simulink model "dq_model"  (R2015a)
settings: Solver=ode45  StartTime=0.0  StopTime=1.5  FixedStep=1e-5  MaxStep=1e-3  RelTol=1e-3
InitFcn:
  | parametriAM
values from neighbouring files (symbols this model uses):
  Imrn = 7.4    [parametriAM.m]
  Ismax = In*sqrt(2)    [parametriAM.m]
  J = 0.019    [parametriAM.m]    (also in podatki.m = 0.01)
  Ki_Imr = 1000    [parametriAM.m]
  Ki_tok = 5.0    (= 5)    [parametriAM.m]
  Ki_wr = 1000    [parametriAM.m]
  Kp_Imr = 100    [parametriAM.m]
  Kp_tok = 0.05    [parametriAM.m]
  Kp_wr = 50    [parametriAM.m]
  Lm = 0.0493    [parametriAM.m]    (also in podatki.m = 0.2342)
  Lr = 0.05315    [parametriAM.m]    (also in podatki.m = 0.2449)
  Ls = 0.05315    [parametriAM.m]    (also in podatki.m = 0.2449)
  Lst = sigma*Ls    (= 0.00742111947319)    [parametriAM.m]
  pp = 3    [parametriAM.m]    (also in podatki.m = 2)
  Rs = 0.594    [parametriAM.m]    (also in podatki.m = 3.7)
  sigma = 1 - 1/((1+sigmaR)*(1+sigmaS))    (= 0.13962595434)    [parametriAM.m]
  Tr = Lr/Rr    (= 0.0771407837446)    [parametriAM.m]
  Udc = Un*sqrt(2)    [parametriAM.m]
  wb_upper_limit_field_weaking = sqrt((Ls^2+Lst^2)/(2*Lst^2*Ls^2))*Usmax/Ismax    [parametriAM.m]
  wn = Udc/sqrt(Ls^2*(Imrn)^2+Lst^2*(Ismax^2-(Imrn)^2))    [maximalnaelipsa.m]    (also in parametriAM.m = Un/sqrt(Ls^2*(Imrn)^2+Lst^2*(Ismax^2-(Imrn)^2))/pp)
libraries: simulink x20
(part 2 of 2)

== system dq_model/motor/Transformacije/Inverzni Park ==
  kot : Inport
  U_dq : Inport  Port=2
  Demux : Demux  Outputs=2
  Mux : Mux  Inputs=2
  "Sum1 " : Sum  Inputs=+-  SaturateOnIntegerOverflow=on  InputSameDT=on  OutDataTypeStr=Inherit: Same as first input
  Sum2 : Sum  SaturateOnIntegerOverflow=on  InputSameDT=on  OutDataTypeStr=Inherit: Same as first input
  cos : Fcn  Expr=cos(u)
  sin : Fcn  Expr=sin(u)
  x_d*cos : Product  SaturateOnIntegerOverflow=on  RndMeth=Zero  InputSameDT=on  OutDataTypeStr=Inherit: Same as first input
  x_d*sin : Product  SaturateOnIntegerOverflow=on  RndMeth=Zero  InputSameDT=on  OutDataTypeStr=Inherit: Same as first input
  x_q*cos : Product  SaturateOnIntegerOverflow=on  RndMeth=Zero  InputSameDT=on  OutDataTypeStr=Inherit: Same as first input
  "x_q*sin " : Product  SaturateOnIntegerOverflow=on  RndMeth=Zero  InputSameDT=on  OutDataTypeStr=Inherit: Same as first input
  U_ab : Outport
  wires:
  Mux/1 -> U_ab/1
  U_dq/1 -> Demux/1
  Demux/1 -> x_d*sin/1, x_d*cos/1
  Demux/2 -> "x_q*sin "/1, x_q*cos/1
  cos/1 -> x_q*cos/2, x_d*cos/2
  sin/1 -> "x_q*sin "/2, x_d*sin/2
  x_d*cos/1 -> "Sum1 "/1
  "x_q*sin "/1 -> "Sum1 "/2
  x_q*cos/1 -> Sum2/2
  x_d*sin/1 -> Sum2/1
  "Sum1 "/1 -> Mux/1
  Sum2/1 -> Mux/2
  kot/1 -> cos/1, sin/1

== system dq_model/motor1/Asinhronski stroj1/Clarke ==
  U_123 : Inport
  ABC_ab1 : Subsystem
  Demux : Demux  Outputs=3
  Mux : Mux  Inputs=2
  U_ab : Outport
  wires:
  U_123/1 -> Demux/1
  Demux/1 -> ABC_ab1/1(A)
  Demux/2 -> ABC_ab1/2(B)
  Demux/3 -> ABC_ab1/3(C)
  ABC_ab1/1(alfa) -> Mux/1
  ABC_ab1/2(beta) -> Mux/2
  Mux/1 -> U_ab/1

== system dq_model/motor1/Asinhronski stroj1/Inverzni Clarke ==
  I_ab : Inport
  Demux : Demux  Outputs=2
  Mux : Mux  Inputs=3
  ab_ABC : Subsystem
  I_123 : Outport
  wires:
  Mux/1 -> I_123/1
  I_ab/1 -> Demux/1
  Demux/1 -> ab_ABC/1(alfa)
  Demux/2 -> ab_ABC/2(beta)
  ab_ABC/1(A) -> Mux/1
  ab_ABC/2(B) -> Mux/2
  ab_ABC/3(C) -> Mux/3

== system dq_model/motor1/Asinhronski stroj1/Inverzni Park ==
  I_dq : Inport
  kot : Inport  Port=2
  Demux : Demux  Outputs=2
  Mux : Mux  Inputs=2
  "Sum1 " : Sum  Inputs=+-  SaturateOnIntegerOverflow=on  InputSameDT=on  OutDataTypeStr=Inherit: Same as first input
  Sum2 : Sum  SaturateOnIntegerOverflow=on  InputSameDT=on  OutDataTypeStr=Inherit: Same as first input
  cos : Fcn  Expr=cos(u)
  sin : Fcn  Expr=sin(u)
  x_d*cos : Product  SaturateOnIntegerOverflow=on  RndMeth=Zero  InputSameDT=on  OutDataTypeStr=Inherit: Same as first input
  x_d*sin : Product  SaturateOnIntegerOverflow=on  RndMeth=Zero  InputSameDT=on  OutDataTypeStr=Inherit: Same as first input
  x_q*cos : Product  SaturateOnIntegerOverflow=on  RndMeth=Zero  InputSameDT=on  OutDataTypeStr=Inherit: Same as first input
  "x_q*sin " : Product  SaturateOnIntegerOverflow=on  RndMeth=Zero  InputSameDT=on  OutDataTypeStr=Inherit: Same as first input
  I_ab : Outport
  wires:
  kot/1 -> sin/1, cos/1
  Sum2/1 -> Mux/2
  "Sum1 "/1 -> Mux/1
  x_d*sin/1 -> Sum2/1
  x_q*cos/1 -> Sum2/2
  "x_q*sin "/1 -> "Sum1 "/2
  x_d*cos/1 -> "Sum1 "/1
  sin/1 -> x_d*sin/2, "x_q*sin "/2
  cos/1 -> x_d*cos/2, x_q*cos/2
  Demux/2 -> x_q*cos/1, "x_q*sin "/1
  Demux/1 -> x_d*cos/1, x_d*sin/1
  I_dq/1 -> Demux/1
  Mux/1 -> I_ab/1

== system dq_model/motor1/Asinhronski stroj1/Mehanika ==
  M_br : Inport
  M_el : Inport  Port=2
  Sum : Sum  Inputs=+-
  eq 2.19 : Subsystem
  wr : Outport
  wires:
  eq 2.19/1(wr) -> wr/1
  M_el/1 -> Sum/1
  Sum/1 -> eq 2.19/1(M)
  M_br/1 -> Sum/2

== system dq_model/motor1/Asinhronski stroj1/Park ==
  U_ab : Inport
  kot : Inport  Port=2
  Demux : Demux  Outputs=2
  Mux : Mux  Inputs=2
  "Sum1 " : Sum  SaturateOnIntegerOverflow=on  InputSameDT=on  OutDataTypeStr=Inherit: Same as first input
  Sum2 : Sum  Inputs=-+  SaturateOnIntegerOverflow=on  InputSameDT=on  OutDataTypeStr=Inherit: Same as first input
  cos : Fcn  Expr=cos(u)
  sin : Fcn  Expr=sin(u)
  x_a*cos : Product  SaturateOnIntegerOverflow=on  RndMeth=Zero  InputSameDT=on  OutDataTypeStr=Inherit: Same as first input
  x_a*sin : Product  SaturateOnIntegerOverflow=on  RndMeth=Zero  InputSameDT=on  OutDataTypeStr=Inherit: Same as first input
  x_b*cos : Product  SaturateOnIntegerOverflow=on  RndMeth=Zero  InputSameDT=on  OutDataTypeStr=Inherit: Same as first input
  "x_b*sin " : Product  SaturateOnIntegerOverflow=on  RndMeth=Zero  InputSameDT=on  OutDataTypeStr=Inherit: Same as first input
  U_dq : Outport
  wires:
  kot/1 -> sin/1, cos/1
  Sum2/1 -> Mux/2
  "Sum1 "/1 -> Mux/1
  x_a*sin/1 -> Sum2/1
  x_b*cos/1 -> Sum2/2
  "x_b*sin "/1 -> "Sum1 "/2
  x_a*cos/1 -> "Sum1 "/1
  sin/1 -> x_a*sin/2, "x_b*sin "/2
  cos/1 -> x_a*cos/2, x_b*cos/2
  Demux/2 -> x_b*cos/1, "x_b*sin "/1
  Demux/1 -> x_a*cos/1, x_a*sin/1
  U_ab/1 -> Demux/1
  Mux/1 -> U_dq/1

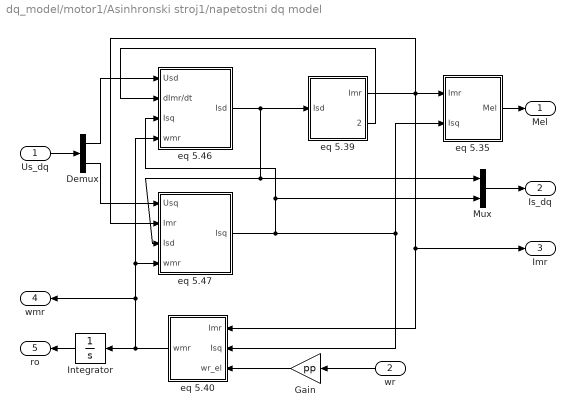
== system dq_model/motor1/Asinhronski stroj1/napetostni dq model ==
  Us_dq : Inport
  wr : Inport  Port=2
  Demux : Demux  Outputs=2
  Gain : Gain  Gain=pp
  Integrator : Integrator
  Mux : Mux  Inputs=2
  eq 5.35 : Subsystem
  eq 5.39 : Subsystem
  eq 5.40 : Subsystem
  eq 5.46 : Subsystem
  eq 5.47 : Subsystem
  Mel : Outport
  Is_dq : Outport  Port=2
  Imr : Outport  Port=3
  wmr : Outport  Port=4
  ro : Outport  Port=5
  wires:
  eq 5.46/1(Isd) -> eq 5.39/1(Isd), eq 5.47/3(Isd), Mux/1
  eq 5.39/2(dImr/dt) -> eq 5.46/2(dImr/dt)
  eq 5.39/1(Imr) -> eq 5.35/1(Imr), eq 5.40/1(Imr), Imr/1, eq 5.47/2(Imr)
  eq 5.47/1(Isq) -> eq 5.35/2(Isq), eq 5.40/2(Isq), eq 5.46/3(Isq), Mux/2
  eq 5.40/1(wmr) -> eq 5.47/4(wmr), eq 5.46/4(wmr), wmr/1, Integrator/1
  eq 5.35/1(Mel) -> Mel/1
  Integrator/1 -> ro/1
  wr/1 -> Gain/1
  Us_dq/1 -> Demux/1
  Demux/1 -> eq 5.46/1(Usd)
  Demux/2 -> eq 5.47/1(Usq)
  Mux/1 -> Is_dq/1
  Gain/1 -> eq 5.40/3(wr_el)

== system dq_model/motor1/Transformacije/Inverzni Clarke ==
  U_ab : Inport
  Demux : Demux  Outputs=2
  Mux : Mux  Inputs=3
  ab_ABC : Subsystem
  U_123 : Outport
  wires:
  Mux/1 -> U_123/1
  U_ab/1 -> Demux/1
  Demux/1 -> ab_ABC/1(alfa)
  Demux/2 -> ab_ABC/2(beta)
  ab_ABC/1(A) -> Mux/1
  ab_ABC/2(B) -> Mux/2
  ab_ABC/3(C) -> Mux/3

== system dq_model/motor1/Transformacije/Inverzni Park ==
  kot : Inport
  U_dq : Inport  Port=2
  Demux : Demux  Outputs=2
  Mux : Mux  Inputs=2
  "Sum1 " : Sum  Inputs=+-  SaturateOnIntegerOverflow=on  InputSameDT=on  OutDataTypeStr=Inherit: Same as first input
  Sum2 : Sum  SaturateOnIntegerOverflow=on  InputSameDT=on  OutDataTypeStr=Inherit: Same as first input
  cos : Fcn  Expr=cos(u)
  sin : Fcn  Expr=sin(u)
  x_d*cos : Product  SaturateOnIntegerOverflow=on  RndMeth=Zero  InputSameDT=on  OutDataTypeStr=Inherit: Same as first input
  x_d*sin : Product  SaturateOnIntegerOverflow=on  RndMeth=Zero  InputSameDT=on  OutDataTypeStr=Inherit: Same as first input
  x_q*cos : Product  SaturateOnIntegerOverflow=on  RndMeth=Zero  InputSameDT=on  OutDataTypeStr=Inherit: Same as first input
  "x_q*sin " : Product  SaturateOnIntegerOverflow=on  RndMeth=Zero  InputSameDT=on  OutDataTypeStr=Inherit: Same as first input
  U_ab : Outport
  wires:
  kot/1 -> sin/1, cos/1
  Sum2/1 -> Mux/2
  "Sum1 "/1 -> Mux/1
  x_d*sin/1 -> Sum2/1
  x_q*cos/1 -> Sum2/2
  "x_q*sin "/1 -> "Sum1 "/2
  x_d*cos/1 -> "Sum1 "/1
  sin/1 -> x_d*sin/2, "x_q*sin "/2
  cos/1 -> x_d*cos/2, x_q*cos/2
  Demux/2 -> x_q*cos/1, "x_q*sin "/1
  Demux/1 -> x_d*cos/1, x_d*sin/1
  U_dq/1 -> Demux/1
  Mux/1 -> U_ab/1

== system dq_model/motor2/Asinhronski stroj1/Clarke ==
  U_123 : Inport
  ABC_ab1 : Subsystem
  Demux : Demux  Outputs=3
  Mux : Mux  Inputs=2
  U_ab : Outport
  wires:
  Mux/1 -> U_ab/1
  ABC_ab1/2(beta) -> Mux/2
  ABC_ab1/1(alfa) -> Mux/1
  Demux/3 -> ABC_ab1/3(C)
  Demux/2 -> ABC_ab1/2(B)
  Demux/1 -> ABC_ab1/1(A)
  U_123/1 -> Demux/1

== system dq_model/motor2/Asinhronski stroj1/Inverzni Clarke ==
  I_ab : Inport
  Demux : Demux  Outputs=2
  Mux : Mux  Inputs=3
  ab_ABC : Subsystem
  I_123 : Outport
  wires:
  ab_ABC/3(C) -> Mux/3
  ab_ABC/2(B) -> Mux/2
  ab_ABC/1(A) -> Mux/1
  Demux/2 -> ab_ABC/2(beta)
  Demux/1 -> ab_ABC/1(alfa)
  I_ab/1 -> Demux/1
  Mux/1 -> I_123/1

== system dq_model/motor2/Asinhronski stroj1/Inverzni Park ==
  I_dq : Inport
  kot : Inport  Port=2
  Demux : Demux  Outputs=2
  Mux : Mux  Inputs=2
  "Sum1 " : Sum  Inputs=+-  SaturateOnIntegerOverflow=on  InputSameDT=on  OutDataTypeStr=Inherit: Same as first input
  Sum2 : Sum  SaturateOnIntegerOverflow=on  InputSameDT=on  OutDataTypeStr=Inherit: Same as first input
  cos : Fcn  Expr=cos(u)
  sin : Fcn  Expr=sin(u)
  x_d*cos : Product  SaturateOnIntegerOverflow=on  RndMeth=Zero  InputSameDT=on  OutDataTypeStr=Inherit: Same as first input
  x_d*sin : Product  SaturateOnIntegerOverflow=on  RndMeth=Zero  InputSameDT=on  OutDataTypeStr=Inherit: Same as first input
  x_q*cos : Product  SaturateOnIntegerOverflow=on  RndMeth=Zero  InputSameDT=on  OutDataTypeStr=Inherit: Same as first input
  "x_q*sin " : Product  SaturateOnIntegerOverflow=on  RndMeth=Zero  InputSameDT=on  OutDataTypeStr=Inherit: Same as first input
  I_ab : Outport
  wires:
  Mux/1 -> I_ab/1
  I_dq/1 -> Demux/1
  Demux/1 -> x_d*sin/1, x_d*cos/1
  Demux/2 -> "x_q*sin "/1, x_q*cos/1
  cos/1 -> x_q*cos/2, x_d*cos/2
  sin/1 -> "x_q*sin "/2, x_d*sin/2
  x_d*cos/1 -> "Sum1 "/1
  "x_q*sin "/1 -> "Sum1 "/2
  x_q*cos/1 -> Sum2/2
  x_d*sin/1 -> Sum2/1
  "Sum1 "/1 -> Mux/1
  Sum2/1 -> Mux/2
  kot/1 -> cos/1, sin/1

== system dq_model/motor2/Asinhronski stroj1/Mehanika ==
  M_br : Inport
  M_el : Inport  Port=2
  Sum : Sum  Inputs=+-
  eq 2.19 : Subsystem
  wr : Outport
  wires:
  M_br/1 -> Sum/2
  Sum/1 -> eq 2.19/1(M)
  M_el/1 -> Sum/1
  eq 2.19/1(wr) -> wr/1

== system dq_model/motor2/Asinhronski stroj1/Park ==
  U_ab : Inport
  kot : Inport  Port=2
  Demux : Demux  Outputs=2
  Mux : Mux  Inputs=2
  "Sum1 " : Sum  SaturateOnIntegerOverflow=on  InputSameDT=on  OutDataTypeStr=Inherit: Same as first input
  Sum2 : Sum  Inputs=-+  SaturateOnIntegerOverflow=on  InputSameDT=on  OutDataTypeStr=Inherit: Same as first input
  cos : Fcn  Expr=cos(u)
  sin : Fcn  Expr=sin(u)
  x_a*cos : Product  SaturateOnIntegerOverflow=on  RndMeth=Zero  InputSameDT=on  OutDataTypeStr=Inherit: Same as first input
  x_a*sin : Product  SaturateOnIntegerOverflow=on  RndMeth=Zero  InputSameDT=on  OutDataTypeStr=Inherit: Same as first input
  x_b*cos : Product  SaturateOnIntegerOverflow=on  RndMeth=Zero  InputSameDT=on  OutDataTypeStr=Inherit: Same as first input
  "x_b*sin " : Product  SaturateOnIntegerOverflow=on  RndMeth=Zero  InputSameDT=on  OutDataTypeStr=Inherit: Same as first input
  U_dq : Outport
  wires:
  Mux/1 -> U_dq/1
  U_ab/1 -> Demux/1
  Demux/1 -> x_a*sin/1, x_a*cos/1
  Demux/2 -> "x_b*sin "/1, x_b*cos/1
  cos/1 -> x_b*cos/2, x_a*cos/2
  sin/1 -> "x_b*sin "/2, x_a*sin/2
  x_a*cos/1 -> "Sum1 "/1
  "x_b*sin "/1 -> "Sum1 "/2
  x_b*cos/1 -> Sum2/2
  x_a*sin/1 -> Sum2/1
  "Sum1 "/1 -> Mux/1
  Sum2/1 -> Mux/2
  kot/1 -> cos/1, sin/1

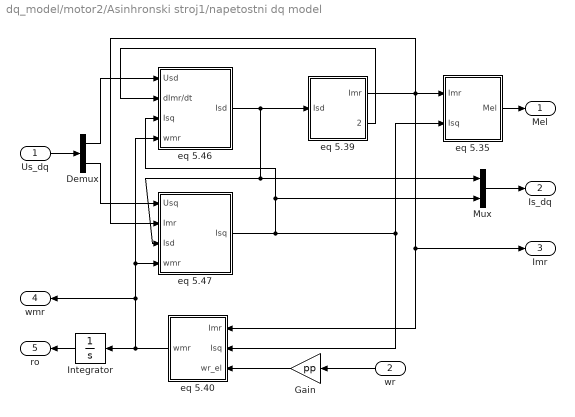
== system dq_model/motor2/Asinhronski stroj1/napetostni dq model ==
  Us_dq : Inport
  wr : Inport  Port=2
  Demux : Demux  Outputs=2
  Gain : Gain  Gain=pp
  Integrator : Integrator
  Mux : Mux  Inputs=2
  eq 5.35 : Subsystem
  eq 5.39 : Subsystem
  eq 5.40 : Subsystem
  eq 5.46 : Subsystem
  eq 5.47 : Subsystem
  Mel : Outport
  Is_dq : Outport  Port=2
  Imr : Outport  Port=3
  wmr : Outport  Port=4
  ro : Outport  Port=5
  wires:
  Gain/1 -> eq 5.40/3(wr_el)
  Mux/1 -> Is_dq/1
  Demux/2 -> eq 5.47/1(Usq)
  Demux/1 -> eq 5.46/1(Usd)
  Us_dq/1 -> Demux/1
  wr/1 -> Gain/1
  Integrator/1 -> ro/1
  eq 5.35/1(Mel) -> Mel/1
  eq 5.40/1(wmr) -> Integrator/1, wmr/1, eq 5.46/4(wmr), eq 5.47/4(wmr)
  eq 5.47/1(Isq) -> Mux/2, eq 5.46/3(Isq), eq 5.40/2(Isq), eq 5.35/2(Isq)
  eq 5.39/1(Imr) -> eq 5.47/2(Imr), Imr/1, eq 5.40/1(Imr), eq 5.35/1(Imr)
  eq 5.39/2(dImr/dt) -> eq 5.46/2(dImr/dt)
  eq 5.46/1(Isd) -> Mux/1, eq 5.47/3(Isd), eq 5.39/1(Isd)

== system dq_model/motor2/Transformacije/Inverzni Clarke ==
  U_ab : Inport
  Demux : Demux  Outputs=2
  Mux : Mux  Inputs=3
  ab_ABC : Subsystem
  U_123 : Outport
  wires:
  ab_ABC/3(C) -> Mux/3
  ab_ABC/2(B) -> Mux/2
  ab_ABC/1(A) -> Mux/1
  Demux/2 -> ab_ABC/2(beta)
  Demux/1 -> ab_ABC/1(alfa)
  U_ab/1 -> Demux/1
  Mux/1 -> U_123/1

== system dq_model/motor2/Transformacije/Inverzni Park ==
  kot : Inport
  U_dq : Inport  Port=2
  Demux : Demux  Outputs=2
  Mux : Mux  Inputs=2
  "Sum1 " : Sum  Inputs=+-  SaturateOnIntegerOverflow=on  InputSameDT=on  OutDataTypeStr=Inherit: Same as first input
  Sum2 : Sum  SaturateOnIntegerOverflow=on  InputSameDT=on  OutDataTypeStr=Inherit: Same as first input
  cos : Fcn  Expr=cos(u)
  sin : Fcn  Expr=sin(u)
  x_d*cos : Product  SaturateOnIntegerOverflow=on  RndMeth=Zero  InputSameDT=on  OutDataTypeStr=Inherit: Same as first input
  x_d*sin : Product  SaturateOnIntegerOverflow=on  RndMeth=Zero  InputSameDT=on  OutDataTypeStr=Inherit: Same as first input
  x_q*cos : Product  SaturateOnIntegerOverflow=on  RndMeth=Zero  InputSameDT=on  OutDataTypeStr=Inherit: Same as first input
  "x_q*sin " : Product  SaturateOnIntegerOverflow=on  RndMeth=Zero  InputSameDT=on  OutDataTypeStr=Inherit: Same as first input
  U_ab : Outport
  wires:
  Mux/1 -> U_ab/1
  U_dq/1 -> Demux/1
  Demux/1 -> x_d*sin/1, x_d*cos/1
  Demux/2 -> "x_q*sin "/1, x_q*cos/1
  cos/1 -> x_q*cos/2, x_d*cos/2
  sin/1 -> "x_q*sin "/2, x_d*sin/2
  x_d*cos/1 -> "Sum1 "/1
  "x_q*sin "/1 -> "Sum1 "/2
  x_q*cos/1 -> Sum2/2
  x_d*sin/1 -> Sum2/1
  "Sum1 "/1 -> Mux/1
  Sum2/1 -> Mux/2
  kot/1 -> cos/1, sin/1

== system dq_model/Tehnika A/Regulacija navora/Limita q toka/Subsystem ==
  High : Inport
  U : Inport  Port=2
  Data Type Duplicate : DataTypeDuplicate  DisableCoverage=on
  Data Type Propagation : simulink/Signal Attributes/Data Type Propagation  PropDataType=fixdt(1, 16)  IfRefDouble=double  IfRefSingle=single  IsSigned=IsSigned1  NumBitsBase=NumBits1  NumBitsMult=1  NumBitsAdd=0  NumBitsAllowFinal=1:128  PropScaling=2^-10  ValuesUsedBestPrec=[5 -7]  SlopeBase=Slope1  SlopeMult=1  SlopeAdd=0  BiasBase=Bias1  BiasMult=1  BiasAdd=0
  Gain : Gain  Gain=-1
  LowerRelop1 : RelationalOperator  DisableCoverage=on  Operator=>  OutDataTypeStr=boolean  ZeroCross=off
  Switch : Switch  Criteria=u2 ~= 0  OutDataTypeStr=Inherit: Inherit via back propagation  ZeroCross=off  SaturateOnIntegerOverflow=on
  Switch2 : Switch  Criteria=u2 ~= 0  OutDataTypeStr=Inherit: Inherit via back propagation  ZeroCross=off  SaturateOnIntegerOverflow=on
  UpperRelop : RelationalOperator  DisableCoverage=on  Operator=<  OutDataTypeStr=boolean
  Uq_lim : Outport
  wires:
  High/1 -> Switch2/1, LowerRelop1/2, Gain/1
  UpperRelop/1 -> Switch/2
  LowerRelop1/1 -> Switch2/2
  Gain/1 -> UpperRelop/2, Switch/1
  Switch/1 -> Data Type Duplicate/2, Switch2/3, Data Type Propagation/3
  Switch2/1 -> Uq_lim/1, Data Type Duplicate/1
  U/1 -> Data Type Propagation/2, Data Type Propagation/1, LowerRelop1/1, Switch/3, UpperRelop/1

== system dq_model/Tehnika A/Regulacija navora/Limita q toka/napetostna limita ==
  Iddej : Inport
  w : Inport  Port=2
  Abs : Abs
  Abs1 : Abs
  Add1 : Sum  Inputs=-+
  Constant : Constant
  Constant1 : Constant  Value=Udc
  Divide : Product  Inputs=*/
  Product2 : Product
  Product3 : Product
  Saturation : Saturate  UpperLimit=1  LowerLimit=0
  Saturation1 : Saturate  UpperLimit=Ismax  LowerLimit=0
  Sqrt : Sqrt  SaturateOnIntegerOverflow=on
  a : Subsystem
  b : Subsystem
  high : Outport
  wires:
  Sqrt/1 -> Product3/1
  Iddej/1 -> Divide/1
  Divide/1 -> Product2/1, Product2/2
  Constant/1 -> Add1/2
  w/1 -> Abs1/1
  Product3/1 -> Abs/1
  Add1/1 -> Sqrt/1
  b/1(b) -> Product3/2
  a/1(a) -> Divide/2
  Abs1/1 -> b/2(w), a/1(w)
  Product2/1 -> Saturation/1
  Saturation/1 -> Add1/1
  Saturation1/1 -> high/1
  Abs/1 -> Saturation1/1
  Constant1/1 -> b/1(U), a/2(U)

== system dq_model/Tehnika A/Regulacija navora/Limita q toka/tokovna ==
  Id : Inport
  Abs : Abs
  Constant : Constant  Value=Ismax^2
  Product1 : Product
  Saturation : Saturate  UpperLimit=Ismax^2  LowerLimit=0
  Scope : Scope  NumInputPorts=2
      settings: TimeRange=auto  MaxDataPoints=5000  SaveToWorkspace=off  SaveName=ScopeData5  YMin=814.57936~-5  YMax=1701.84674~5  SampleTime=-1
  Sqrt : Sqrt  SaturateOnIntegerOverflow=on
  Subtract : Sum  Inputs=+-
  high : Outport
  wires:
  Sqrt/1 -> Abs/1
  Id/1 -> Product1/2, Product1/1
  Constant/1 -> Subtract/1
  Product1/1 -> Subtract/2
  Abs/1 -> high/1
  Subtract/1 -> Scope/1, Saturation/1
  Saturation/1 -> Scope/2, Sqrt/1

== system dq_model/Tehnika A/Tok regulator/Limita Uq/Subsystem ==
  High : Inport
  U : Inport  Port=2
  Data Type Duplicate : DataTypeDuplicate  DisableCoverage=on
  Data Type Propagation : simulink/Signal Attributes/Data Type Propagation  PropDataType=fixdt(1, 16)  IfRefDouble=double  IfRefSingle=single  IsSigned=IsSigned1  NumBitsBase=NumBits1  NumBitsMult=1  NumBitsAdd=0  NumBitsAllowFinal=1:128  PropScaling=2^-10  ValuesUsedBestPrec=[5 -7]  SlopeBase=Slope1  SlopeMult=1  SlopeAdd=0  BiasBase=Bias1  BiasMult=1  BiasAdd=0
  Gain : Gain  Gain=-1
  LowerRelop1 : RelationalOperator  DisableCoverage=on  Operator=>  OutDataTypeStr=boolean  ZeroCross=off
  Switch : Switch  Criteria=u2 ~= 0  OutDataTypeStr=Inherit: Inherit via back propagation  ZeroCross=off  SaturateOnIntegerOverflow=on
  Switch2 : Switch  Criteria=u2 ~= 0  OutDataTypeStr=Inherit: Inherit via back propagation  ZeroCross=off  SaturateOnIntegerOverflow=on
  UpperRelop : RelationalOperator  DisableCoverage=on  Operator=<  OutDataTypeStr=boolean
  Uq_lim : Outport
  wires:
  High/1 -> Switch2/1, LowerRelop1/2, Gain/1
  UpperRelop/1 -> Switch/2
  LowerRelop1/1 -> Switch2/2
  Gain/1 -> UpperRelop/2, Switch/1
  Switch/1 -> Data Type Duplicate/2, Switch2/3, Data Type Propagation/3
  Switch2/1 -> Uq_lim/1, Data Type Duplicate/1
  U/1 -> Data Type Propagation/2, Data Type Propagation/1, LowerRelop1/1, Switch/3, UpperRelop/1

== system dq_model/Tehnika B/Regulacija navora/Limita q toka/Subsystem ==
  High : Inport
  U : Inport  Port=2
  Data Type Duplicate : DataTypeDuplicate  DisableCoverage=on
  Data Type Propagation : simulink/Signal Attributes/Data Type Propagation  PropDataType=fixdt(1, 16)  IfRefDouble=double  IfRefSingle=single  IsSigned=IsSigned1  NumBitsBase=NumBits1  NumBitsMult=1  NumBitsAdd=0  NumBitsAllowFinal=1:128  PropScaling=2^-10  ValuesUsedBestPrec=[5 -7]  SlopeBase=Slope1  SlopeMult=1  SlopeAdd=0  BiasBase=Bias1  BiasMult=1  BiasAdd=0
  Gain : Gain  Gain=-1
  LowerRelop1 : RelationalOperator  DisableCoverage=on  Operator=>  OutDataTypeStr=boolean  ZeroCross=off
  Switch : Switch  Criteria=u2 ~= 0  OutDataTypeStr=Inherit: Inherit via back propagation  ZeroCross=off  SaturateOnIntegerOverflow=on
  Switch2 : Switch  Criteria=u2 ~= 0  OutDataTypeStr=Inherit: Inherit via back propagation  ZeroCross=off  SaturateOnIntegerOverflow=on
  UpperRelop : RelationalOperator  DisableCoverage=on  Operator=<  OutDataTypeStr=boolean
  Uq_lim : Outport
  wires:
  High/1 -> Switch2/1, LowerRelop1/2, Gain/1
  UpperRelop/1 -> Switch/2
  LowerRelop1/1 -> Switch2/2
  Gain/1 -> UpperRelop/2, Switch/1
  Switch/1 -> Data Type Duplicate/2, Switch2/3, Data Type Propagation/3
  Switch2/1 -> Uq_lim/1, Data Type Duplicate/1
  U/1 -> Data Type Propagation/2, Data Type Propagation/1, LowerRelop1/1, Switch/3, UpperRelop/1

== system dq_model/Tehnika B/Regulacija navora/Limita q toka/napetostna limita ==
  Iddej : Inport
  w : Inport  Port=2
  Abs : Abs
  Abs1 : Abs
  Add1 : Sum  Inputs=-+
  Constant : Constant
  Constant1 : Constant  Value=Udc
  Divide : Product  Inputs=*/
  Product2 : Product
  Product3 : Product
  Saturation : Saturate  UpperLimit=1  LowerLimit=0
  Saturation1 : Saturate  UpperLimit=Ismax  LowerLimit=0
  Sqrt : Sqrt  SaturateOnIntegerOverflow=on
  a : Subsystem
  b : Subsystem
  high : Outport
  wires:
  Constant1/1 -> a/2(U), b/1(U)
  Abs/1 -> Saturation1/1
  Saturation1/1 -> high/1
  Saturation/1 -> Add1/1
  Product2/1 -> Saturation/1
  Abs1/1 -> a/1(w), b/2(w)
  a/1(a) -> Divide/2
  b/1(b) -> Product3/2
  Add1/1 -> Sqrt/1
  Product3/1 -> Abs/1
  w/1 -> Abs1/1
  Constant/1 -> Add1/2
  Divide/1 -> Product2/2, Product2/1
  Iddej/1 -> Divide/1
  Sqrt/1 -> Product3/1

== system dq_model/Tehnika B/Regulacija navora/Limita q toka/tokovna ==
  Id : Inport
  Abs : Abs
  Constant : Constant  Value=Ismax^2
  Product1 : Product
  Saturation : Saturate  UpperLimit=Ismax^2  LowerLimit=0
  Scope : Scope  NumInputPorts=2
      settings: TimeRange=auto  MaxDataPoints=5000  SaveToWorkspace=off  SaveName=ScopeData5  YMin=814.57936~-5  YMax=1701.84674~5  SampleTime=-1
  Sqrt : Sqrt  SaturateOnIntegerOverflow=on
  Subtract : Sum  Inputs=+-
  high : Outport
  wires:
  Saturation/1 -> Sqrt/1, Scope/2
  Subtract/1 -> Saturation/1, Scope/1
  Abs/1 -> high/1
  Product1/1 -> Subtract/2
  Constant/1 -> Subtract/1
  Id/1 -> Product1/1, Product1/2
  Sqrt/1 -> Abs/1

== system dq_model/Tehnika B/Tok regulator/Limita Uq/Subsystem ==
  High : Inport
  U : Inport  Port=2
  Data Type Duplicate : DataTypeDuplicate  DisableCoverage=on
  Data Type Propagation : simulink/Signal Attributes/Data Type Propagation  PropDataType=fixdt(1, 16)  IfRefDouble=double  IfRefSingle=single  IsSigned=IsSigned1  NumBitsBase=NumBits1  NumBitsMult=1  NumBitsAdd=0  NumBitsAllowFinal=1:128  PropScaling=2^-10  ValuesUsedBestPrec=[5 -7]  SlopeBase=Slope1  SlopeMult=1  SlopeAdd=0  BiasBase=Bias1  BiasMult=1  BiasAdd=0
  Gain : Gain  Gain=-1
  LowerRelop1 : RelationalOperator  DisableCoverage=on  Operator=>  OutDataTypeStr=boolean  ZeroCross=off
  Switch : Switch  Criteria=u2 ~= 0  OutDataTypeStr=Inherit: Inherit via back propagation  ZeroCross=off  SaturateOnIntegerOverflow=on
  Switch2 : Switch  Criteria=u2 ~= 0  OutDataTypeStr=Inherit: Inherit via back propagation  ZeroCross=off  SaturateOnIntegerOverflow=on
  UpperRelop : RelationalOperator  DisableCoverage=on  Operator=<  OutDataTypeStr=boolean
  Uq_lim : Outport
  wires:
  High/1 -> Switch2/1, LowerRelop1/2, Gain/1
  UpperRelop/1 -> Switch/2
  LowerRelop1/1 -> Switch2/2
  Gain/1 -> UpperRelop/2, Switch/1
  Switch/1 -> Data Type Duplicate/2, Switch2/3, Data Type Propagation/3
  Switch2/1 -> Uq_lim/1, Data Type Duplicate/1
  U/1 -> Data Type Propagation/2, Data Type Propagation/1, LowerRelop1/1, Switch/3, UpperRelop/1

== system dq_model/Tehnika s/Regulacija navora/Limita q toka/napetostna limita ==
  Iddej : Inport
  w : Inport  Port=2
  Abs : Abs
  Abs1 : Abs
  Add1 : Sum  Inputs=-+
  Constant : Constant
  Constant1 : Constant  Value=Udc
  Divide : Product  Inputs=*/
  Product2 : Product
  Product3 : Product
  Saturation : Saturate  UpperLimit=1  LowerLimit=0
  Saturation1 : Saturate  UpperLimit=Ismax  LowerLimit=0
  Sqrt : Sqrt  SaturateOnIntegerOverflow=on
  a : Subsystem
  b : Subsystem
  high : Outport
  wires:
  Constant1/1 -> a/2(U), b/1(U)
  Abs/1 -> Saturation1/1
  Saturation1/1 -> high/1
  Saturation/1 -> Add1/1
  Product2/1 -> Saturation/1
  Abs1/1 -> a/1(w), b/2(w)
  a/1(a) -> Divide/2
  b/1(b) -> Product3/2
  Add1/1 -> Sqrt/1
  Product3/1 -> Abs/1
  w/1 -> Abs1/1
  Constant/1 -> Add1/2
  Divide/1 -> Product2/2, Product2/1
  Iddej/1 -> Divide/1
  Sqrt/1 -> Product3/1

== system dq_model/Tehnika s/Regulacija navora/Limita q toka/tokovna ==
  Id : Inport
  Abs : Abs
  Constant : Constant  Value=Ismax^2
  Product1 : Product
  Saturation : Saturate  UpperLimit=Ismax^2  LowerLimit=0
  Scope : Scope  NumInputPorts=2
      settings: TimeRange=auto  MaxDataPoints=5000  SaveToWorkspace=off  SaveName=ScopeData5  YMin=814.57936~-5  YMax=1701.84674~5  SampleTime=-1
  Sqrt : Sqrt  SaturateOnIntegerOverflow=on
  Subtract : Sum  Inputs=+-
  high : Outport
  wires:
  Saturation/1 -> Sqrt/1, Scope/2
  Subtract/1 -> Saturation/1, Scope/1
  Abs/1 -> high/1
  Product1/1 -> Subtract/2
  Constant/1 -> Subtract/1
  Id/1 -> Product1/1, Product1/2
  Sqrt/1 -> Abs/1

== system dq_model/Tehnika s/Tok regulator/Limita Uq/Subsystem ==
  High : Inport
  U : Inport  Port=2
  Data Type Duplicate : DataTypeDuplicate  DisableCoverage=on
  Data Type Propagation : simulink/Signal Attributes/Data Type Propagation  PropDataType=fixdt(1, 16)  IfRefDouble=double  IfRefSingle=single  IsSigned=IsSigned1  NumBitsBase=NumBits1  NumBitsMult=1  NumBitsAdd=0  NumBitsAllowFinal=1:128  PropScaling=2^-10  ValuesUsedBestPrec=[5 -7]  SlopeBase=Slope1  SlopeMult=1  SlopeAdd=0  BiasBase=Bias1  BiasMult=1  BiasAdd=0
  Gain : Gain  Gain=-1
  LowerRelop1 : RelationalOperator  DisableCoverage=on  Operator=>  OutDataTypeStr=boolean  ZeroCross=off
  Switch : Switch  Criteria=u2 ~= 0  OutDataTypeStr=Inherit: Inherit via back propagation  ZeroCross=off  SaturateOnIntegerOverflow=on
  Switch2 : Switch  Criteria=u2 ~= 0  OutDataTypeStr=Inherit: Inherit via back propagation  ZeroCross=off  SaturateOnIntegerOverflow=on
  UpperRelop : RelationalOperator  DisableCoverage=on  Operator=<  OutDataTypeStr=boolean  ZeroCross=off
  Uq_lim : Outport
  wires:
  High/1 -> Switch2/1, LowerRelop1/2, Gain/1
  UpperRelop/1 -> Switch/2
  LowerRelop1/1 -> Switch2/2
  Gain/1 -> UpperRelop/2, Switch/1
  Switch/1 -> Data Type Duplicate/2, Switch2/3, Data Type Propagation/3
  Switch2/1 -> Uq_lim/1, Data Type Duplicate/1
  U/1 -> Data Type Propagation/2, Data Type Propagation/1, LowerRelop1/1, Switch/3, UpperRelop/1

== system dq_model/motor/Asinhronski stroj1/Clarke/ABC_ab1 ==
  A : Inport
  B : Inport  Port=2
  C : Inport  Port=3
  Gain1 : Gain  Gain=2
  Gain2 : Gain
  Gain24 : Gain  Gain=sqrt(3)/3
  Sum11 : Sum
  Terminator : Terminator
  alfa : Outport
  beta : Outport  Port=2
  wires:
  C/1 -> Terminator/1
  Gain1/1 -> Sum11/2
  B/1 -> Gain1/1
  Gain24/1 -> beta/1
  Gain2/1 -> alfa/1
  Sum11/1 -> Gain24/1
  A/1 -> Sum11/1, Gain2/1

== system dq_model/motor/Asinhronski stroj1/Inverzni Clarke/ab_ABC ==
  alfa : Inport
  beta : Inport  Port=2
  Gain1 : Gain
  Gain2 : Gain  Gain=-0.5
  Gain25 : Gain  Gain=sqrt(3)/2
  Gain3 : Gain  Gain=sqrt(3)/2
  Gain4 : Gain  Gain=0.5
  Sum10 : Sum
  Sum11 : Sum  Inputs=--
  A : Outport
  B : Outport  Port=2
  C : Outport  Port=3
  wires:
  Gain3/1 -> Sum11/2
  beta/1 -> Gain25/1, Gain3/1
  Gain4/1 -> Sum11/1
  Gain25/1 -> Sum10/2
  Gain2/1 -> Sum10/1
  alfa/1 -> Gain1/1, Gain2/1, Gain4/1
  Gain1/1 -> A/1
  Sum10/1 -> B/1
  Sum11/1 -> C/1

== system dq_model/motor/Asinhronski stroj1/Mehanika/eq 2.19 ==
  M : Inport
  Gain1 : Gain  Gain=1/J
  Integrator : Integrator
  wr : Outport
  wires:
  Integrator/1 -> wr/1
  M/1 -> Gain1/1
  Gain1/1 -> Integrator/1

== system dq_model/motor/Asinhronski stroj1/napetostni dq model/eq 5.35 ==
  Imr : Inport
  Isq : Inport  Port=2
  Gain : Gain  Gain=3*pp/2
  Gain2 : Gain  Gain=Lm*Lm/Lr
  Product : Product  RndMeth=Zero
  Mel : Outport
  wires:
  Gain/1 -> Gain2/1
  Gain2/1 -> Mel/1
  Product/1 -> Gain/1
  Isq/1 -> Product/2
  Imr/1 -> Product/1

== system dq_model/motor/Asinhronski stroj1/napetostni dq model/eq 5.39 ==
  Isd : Inport
  Gain : Gain  Gain=1/Tr
  Integrator : Integrator  InitialCondition=1e-3
  Sum : Sum  Inputs=|+-
  Imr : Outport
  dImr/dt : Outport  Port=2
  wires:
  Gain/1 -> dImr/dt/1, Integrator/1
  Sum/1 -> Gain/1
  Integrator/1 -> Sum/2, Imr/1
  Isd/1 -> Sum/1

== system dq_model/motor/Asinhronski stroj1/napetostni dq model/eq 5.40 ==
  Imr : Inport
  Isq : Inport  Port=2
  wr_el : Inport  Port=3
  Divide : Product  Inputs=*/
  Gain2 : Gain  Gain=Tr
  Saturation : Saturate  UpperLimit=2*pi*50  LowerLimit=-2*pi*50
  Sum : Sum  Inputs=|++
  wmr : Outport
  wires:
  Saturation/1 -> Sum/1
  Sum/1 -> wmr/1
  wr_el/1 -> Sum/2
  Divide/1 -> Saturation/1  "ws"
  Gain2/1 -> Divide/2
  Imr/1 -> Gain2/1
  Isq/1 -> Divide/1

== system dq_model/motor/Asinhronski stroj1/napetostni dq model/eq 5.46 ==
  Usd : Inport
  dImr/dt : Inport  Port=2
  Isq : Inport  Port=3
  wmr : Inport  Port=4
  Gain : Gain  Gain=1/(sigma*Ls)
  Gain1 : Gain  Gain=Rs
  Gain2 : Gain  Gain=(1-sigma)*Ls
  Gain3 : Gain  Gain=sigma*Ls
  Integrator : Integrator
  Product : Product  RndMeth=Zero
  Sum : Sum  Inputs=+--+
  Isd : Outport
  wires:
  Gain3/1 -> Sum/4
  Product/1 -> Gain3/1
  Isq/1 -> Product/1
  wmr/1 -> Product/2
  Gain2/1 -> Sum/3
  dImr/dt/1 -> Gain2/1
  Gain1/1 -> Sum/2
  Usd/1 -> Sum/1
  Sum/1 -> Gain/1
  Gain/1 -> Integrator/1
  Integrator/1 -> Gain1/1, Isd/1

== system dq_model/motor/Asinhronski stroj1/napetostni dq model/eq 5.47 ==
  Usq : Inport
  Imr : Inport  Port=2
  Isd : Inport  Port=3
  wmr : Inport  Port=4
  Gain : Gain  Gain=1/(sigma*Ls)
  Gain1 : Gain  Gain=Rs
  Gain2 : Gain  Gain=(1-sigma)*Ls
  Gain3 : Gain  Gain=sigma*Ls
  Integrator : Integrator
  Product : Product  RndMeth=Zero
  Product1 : Product  RndMeth=Zero
  Sum : Sum  Inputs=+---
  Isq : Outport
  wires:
  Gain3/1 -> Sum/4
  Product1/1 -> Gain3/1
  Isd/1 -> Product1/2
  Gain2/1 -> Sum/3
  Product/1 -> Gain2/1
  wmr/1 -> Product1/1, Product/2
  Imr/1 -> Product/1
  Gain1/1 -> Sum/2
  Usq/1 -> Sum/1
  Sum/1 -> Gain/1
  Gain/1 -> Integrator/1
  Integrator/1 -> Gain1/1, Isq/1

== system dq_model/motor/Transformacije/Inverzni Clarke/ab_ABC ==
  alfa : Inport
  beta : Inport  Port=2
  Gain1 : Gain
  Gain2 : Gain  Gain=-0.5
  Gain25 : Gain  Gain=sqrt(3)/2
  Gain3 : Gain  Gain=sqrt(3)/2
  Gain4 : Gain  Gain=0.5
  Sum10 : Sum
  Sum11 : Sum  Inputs=--
  A : Outport
  B : Outport  Port=2
  C : Outport  Port=3
  wires:
  Gain3/1 -> Sum11/2
  beta/1 -> Gain25/1, Gain3/1
  Gain4/1 -> Sum11/1
  Gain25/1 -> Sum10/2
  Gain2/1 -> Sum10/1
  alfa/1 -> Gain1/1, Gain2/1, Gain4/1
  Gain1/1 -> A/1
  Sum10/1 -> B/1
  Sum11/1 -> C/1

== system dq_model/motor1/Asinhronski stroj1/Clarke/ABC_ab1 ==
  A : Inport
  B : Inport  Port=2
  C : Inport  Port=3
  Gain1 : Gain  Gain=2
  Gain2 : Gain
  Gain24 : Gain  Gain=sqrt(3)/3
  Sum11 : Sum
  Terminator : Terminator
  alfa : Outport
  beta : Outport  Port=2
  wires:
  A/1 -> Gain2/1, Sum11/1
  Sum11/1 -> Gain24/1
  Gain2/1 -> alfa/1
  Gain24/1 -> beta/1
  B/1 -> Gain1/1
  Gain1/1 -> Sum11/2
  C/1 -> Terminator/1

== system dq_model/motor1/Asinhronski stroj1/Inverzni Clarke/ab_ABC ==
  alfa : Inport
  beta : Inport  Port=2
  Gain1 : Gain
  Gain2 : Gain  Gain=-0.5
  Gain25 : Gain  Gain=sqrt(3)/2
  Gain3 : Gain  Gain=sqrt(3)/2
  Gain4 : Gain  Gain=0.5
  Sum10 : Sum
  Sum11 : Sum  Inputs=--
  A : Outport
  B : Outport  Port=2
  C : Outport  Port=3
  wires:
  Sum11/1 -> C/1
  Sum10/1 -> B/1
  Gain1/1 -> A/1
  alfa/1 -> Gain4/1, Gain2/1, Gain1/1
  Gain2/1 -> Sum10/1
  Gain25/1 -> Sum10/2
  Gain4/1 -> Sum11/1
  beta/1 -> Gain3/1, Gain25/1
  Gain3/1 -> Sum11/2

== system dq_model/motor1/Asinhronski stroj1/Mehanika/eq 2.19 ==
  M : Inport
  Gain1 : Gain  Gain=1/J
  Integrator : Integrator
  wr : Outport
  wires:
  Gain1/1 -> Integrator/1
  M/1 -> Gain1/1
  Integrator/1 -> wr/1

== system dq_model/motor1/Asinhronski stroj1/napetostni dq model/eq 5.35 ==
  Imr : Inport
  Isq : Inport  Port=2
  Gain : Gain  Gain=3*pp/2
  Gain2 : Gain  Gain=Lm*Lm/Lr
  Product : Product  RndMeth=Zero
  Mel : Outport
  wires:
  Imr/1 -> Product/1
  Isq/1 -> Product/2
  Product/1 -> Gain/1
  Gain2/1 -> Mel/1
  Gain/1 -> Gain2/1

== system dq_model/motor1/Asinhronski stroj1/napetostni dq model/eq 5.39 ==
  Isd : Inport
  Gain : Gain  Gain=1/Tr
  Integrator : Integrator  InitialCondition=1e-3
  Sum : Sum  Inputs=|+-
  Imr : Outport
  dImr/dt : Outport  Port=2
  wires:
  Isd/1 -> Sum/1
  Integrator/1 -> Imr/1, Sum/2
  Sum/1 -> Gain/1
  Gain/1 -> Integrator/1, dImr/dt/1

== system dq_model/motor1/Asinhronski stroj1/napetostni dq model/eq 5.40 ==
  Imr : Inport
  Isq : Inport  Port=2
  wr_el : Inport  Port=3
  Divide : Product  Inputs=*/
  Gain2 : Gain  Gain=Tr
  Saturation : Saturate  UpperLimit=2*pi*50  LowerLimit=-2*pi*50
  Sum : Sum  Inputs=|++
  wmr : Outport
  wires:
  Isq/1 -> Divide/1
  Imr/1 -> Gain2/1
  Gain2/1 -> Divide/2
  Divide/1 -> Saturation/1  "ws"
  wr_el/1 -> Sum/2
  Sum/1 -> wmr/1
  Saturation/1 -> Sum/1

== system dq_model/motor1/Asinhronski stroj1/napetostni dq model/eq 5.46 ==
  Usd : Inport
  dImr/dt : Inport  Port=2
  Isq : Inport  Port=3
  wmr : Inport  Port=4
  Gain : Gain  Gain=1/(sigma*Ls)
  Gain1 : Gain  Gain=Rs
  Gain2 : Gain  Gain=(1-sigma)*Ls
  Gain3 : Gain  Gain=sigma*Ls
  Integrator : Integrator
  Product : Product  RndMeth=Zero
  Sum : Sum  Inputs=+--+
  Isd : Outport
  wires:
  Integrator/1 -> Isd/1, Gain1/1
  Gain/1 -> Integrator/1
  Sum/1 -> Gain/1
  Usd/1 -> Sum/1
  Gain1/1 -> Sum/2
  dImr/dt/1 -> Gain2/1
  Gain2/1 -> Sum/3
  wmr/1 -> Product/2
  Isq/1 -> Product/1
  Product/1 -> Gain3/1
  Gain3/1 -> Sum/4

== system dq_model/motor1/Asinhronski stroj1/napetostni dq model/eq 5.47 ==
  Usq : Inport
  Imr : Inport  Port=2
  Isd : Inport  Port=3
  wmr : Inport  Port=4
  Gain : Gain  Gain=1/(sigma*Ls)
  Gain1 : Gain  Gain=Rs
  Gain2 : Gain  Gain=(1-sigma)*Ls
  Gain3 : Gain  Gain=sigma*Ls
  Integrator : Integrator
  Product : Product  RndMeth=Zero
  Product1 : Product  RndMeth=Zero
  Sum : Sum  Inputs=+---
  Isq : Outport
  wires:
  Integrator/1 -> Isq/1, Gain1/1
  Gain/1 -> Integrator/1
  Sum/1 -> Gain/1
  Usq/1 -> Sum/1
  Gain1/1 -> Sum/2
  Imr/1 -> Product/1
  wmr/1 -> Product/2, Product1/1
  Product/1 -> Gain2/1
  Gain2/1 -> Sum/3
  Isd/1 -> Product1/2
  Product1/1 -> Gain3/1
  Gain3/1 -> Sum/4

== system dq_model/motor1/Transformacije/Inverzni Clarke/ab_ABC ==
  alfa : Inport
  beta : Inport  Port=2
  Gain1 : Gain
  Gain2 : Gain  Gain=-0.5
  Gain25 : Gain  Gain=sqrt(3)/2
  Gain3 : Gain  Gain=sqrt(3)/2
  Gain4 : Gain  Gain=0.5
  Sum10 : Sum
  Sum11 : Sum  Inputs=--
  A : Outport
  B : Outport  Port=2
  C : Outport  Port=3
  wires:
  Sum11/1 -> C/1
  Sum10/1 -> B/1
  Gain1/1 -> A/1
  alfa/1 -> Gain4/1, Gain2/1, Gain1/1
  Gain2/1 -> Sum10/1
  Gain25/1 -> Sum10/2
  Gain4/1 -> Sum11/1
  beta/1 -> Gain3/1, Gain25/1
  Gain3/1 -> Sum11/2

== system dq_model/motor2/Asinhronski stroj1/Clarke/ABC_ab1 ==
  A : Inport
  B : Inport  Port=2
  C : Inport  Port=3
  Gain1 : Gain  Gain=2
  Gain2 : Gain
  Gain24 : Gain  Gain=sqrt(3)/3
  Sum11 : Sum
  Terminator : Terminator
  alfa : Outport
  beta : Outport  Port=2
  wires:
  C/1 -> Terminator/1
  Gain1/1 -> Sum11/2
  B/1 -> Gain1/1
  Gain24/1 -> beta/1
  Gain2/1 -> alfa/1
  Sum11/1 -> Gain24/1
  A/1 -> Sum11/1, Gain2/1

== system dq_model/motor2/Asinhronski stroj1/Inverzni Clarke/ab_ABC ==
  alfa : Inport
  beta : Inport  Port=2
  Gain1 : Gain
  Gain2 : Gain  Gain=-0.5
  Gain25 : Gain  Gain=sqrt(3)/2
  Gain3 : Gain  Gain=sqrt(3)/2
  Gain4 : Gain  Gain=0.5
  Sum10 : Sum
  Sum11 : Sum  Inputs=--
  A : Outport
  B : Outport  Port=2
  C : Outport  Port=3
  wires:
  Gain3/1 -> Sum11/2
  beta/1 -> Gain25/1, Gain3/1
  Gain4/1 -> Sum11/1
  Gain25/1 -> Sum10/2
  Gain2/1 -> Sum10/1
  alfa/1 -> Gain1/1, Gain2/1, Gain4/1
  Gain1/1 -> A/1
  Sum10/1 -> B/1
  Sum11/1 -> C/1

== system dq_model/motor2/Asinhronski stroj1/Mehanika/eq 2.19 ==
  M : Inport
  Gain1 : Gain  Gain=1/J
  Integrator : Integrator
  wr : Outport
  wires:
  Integrator/1 -> wr/1
  M/1 -> Gain1/1
  Gain1/1 -> Integrator/1

== system dq_model/motor2/Asinhronski stroj1/napetostni dq model/eq 5.35 ==
  Imr : Inport
  Isq : Inport  Port=2
  Gain : Gain  Gain=3*pp/2
  Gain2 : Gain  Gain=Lm*Lm/Lr
  Product : Product  RndMeth=Zero
  Mel : Outport
  wires:
  Gain/1 -> Gain2/1
  Gain2/1 -> Mel/1
  Product/1 -> Gain/1
  Isq/1 -> Product/2
  Imr/1 -> Product/1

== system dq_model/motor2/Asinhronski stroj1/napetostni dq model/eq 5.39 ==
  Isd : Inport
  Gain : Gain  Gain=1/Tr
  Integrator : Integrator  InitialCondition=1e-3
  Sum : Sum  Inputs=|+-
  Imr : Outport
  dImr/dt : Outport  Port=2
  wires:
  Gain/1 -> dImr/dt/1, Integrator/1
  Sum/1 -> Gain/1
  Integrator/1 -> Sum/2, Imr/1
  Isd/1 -> Sum/1

== system dq_model/motor2/Asinhronski stroj1/napetostni dq model/eq 5.40 ==
  Imr : Inport
  Isq : Inport  Port=2
  wr_el : Inport  Port=3
  Divide : Product  Inputs=*/
  Gain2 : Gain  Gain=Tr
  Saturation : Saturate  UpperLimit=2*pi*50  LowerLimit=-2*pi*50
  Sum : Sum  Inputs=|++
  wmr : Outport
  wires:
  Saturation/1 -> Sum/1
  Sum/1 -> wmr/1
  wr_el/1 -> Sum/2
  Divide/1 -> Saturation/1  "ws"
  Gain2/1 -> Divide/2
  Imr/1 -> Gain2/1
  Isq/1 -> Divide/1

== system dq_model/motor2/Asinhronski stroj1/napetostni dq model/eq 5.46 ==
  Usd : Inport
  dImr/dt : Inport  Port=2
  Isq : Inport  Port=3
  wmr : Inport  Port=4
  Gain : Gain  Gain=1/(sigma*Ls)
  Gain1 : Gain  Gain=Rs
  Gain2 : Gain  Gain=(1-sigma)*Ls
  Gain3 : Gain  Gain=sigma*Ls
  Integrator : Integrator
  Product : Product  RndMeth=Zero
  Sum : Sum  Inputs=+--+
  Isd : Outport
  wires:
  Gain3/1 -> Sum/4
  Product/1 -> Gain3/1
  Isq/1 -> Product/1
  wmr/1 -> Product/2
  Gain2/1 -> Sum/3
  dImr/dt/1 -> Gain2/1
  Gain1/1 -> Sum/2
  Usd/1 -> Sum/1
  Sum/1 -> Gain/1
  Gain/1 -> Integrator/1
  Integrator/1 -> Gain1/1, Isd/1

== system dq_model/motor2/Asinhronski stroj1/napetostni dq model/eq 5.47 ==
  Usq : Inport
  Imr : Inport  Port=2
  Isd : Inport  Port=3
  wmr : Inport  Port=4
  Gain : Gain  Gain=1/(sigma*Ls)
  Gain1 : Gain  Gain=Rs
  Gain2 : Gain  Gain=(1-sigma)*Ls
  Gain3 : Gain  Gain=sigma*Ls
  Integrator : Integrator
  Product : Product  RndMeth=Zero
  Product1 : Product  RndMeth=Zero
  Sum : Sum  Inputs=+---
  Isq : Outport
  wires:
  Gain3/1 -> Sum/4
  Product1/1 -> Gain3/1
  Isd/1 -> Product1/2
  Gain2/1 -> Sum/3
  Product/1 -> Gain2/1
  wmr/1 -> Product1/1, Product/2
  Imr/1 -> Product/1
  Gain1/1 -> Sum/2
  Usq/1 -> Sum/1
  Sum/1 -> Gain/1
  Gain/1 -> Integrator/1
  Integrator/1 -> Gain1/1, Isq/1

== system dq_model/motor2/Transformacije/Inverzni Clarke/ab_ABC ==
  alfa : Inport
  beta : Inport  Port=2
  Gain1 : Gain
  Gain2 : Gain  Gain=-0.5
  Gain25 : Gain  Gain=sqrt(3)/2
  Gain3 : Gain  Gain=sqrt(3)/2
  Gain4 : Gain  Gain=0.5
  Sum10 : Sum
  Sum11 : Sum  Inputs=--
  A : Outport
  B : Outport  Port=2
  C : Outport  Port=3
  wires:
  Gain3/1 -> Sum11/2
  beta/1 -> Gain25/1, Gain3/1
  Gain4/1 -> Sum11/1
  Gain25/1 -> Sum10/2
  Gain2/1 -> Sum10/1
  alfa/1 -> Gain1/1, Gain2/1, Gain4/1
  Gain1/1 -> A/1
  Sum10/1 -> B/1
  Sum11/1 -> C/1

== system dq_model/Tehnika A/Regulacija navora/Limita q toka/napetostna limita/a ==
  w : Inport
  U : Inport  Port=2
  Add3 : Sum
  Constant2 : Constant  Value=0.001
  Divide : Product  Inputs=*/
  Gain : Gain  Gain=1/Ls
  a : Outport
  wires:
  Gain/1 -> Divide/1
  Constant2/1 -> Add3/2
  Add3/1 -> Divide/2
  w/1 -> Add3/1
  Divide/1 -> a/1
  U/1 -> Gain/1

== system dq_model/Tehnika A/Regulacija navora/Limita q toka/napetostna limita/b ==
  U : Inport
  w : Inport  Port=2
  Add4 : Sum
  Constant4 : Constant  Value=0.001
  Divide1 : Product  Inputs=*/
  Gain : Gain  Gain=1/Lst
  b : Outport
  wires:
  Divide1/1 -> b/1
  w/1 -> Add4/1
  Add4/1 -> Divide1/2
  Constant4/1 -> Add4/2
  U/1 -> Gain/1
  Gain/1 -> Divide1/1

== system dq_model/Tehnika B/Regulacija navora/Limita q toka/napetostna limita/a ==
  w : Inport
  U : Inport  Port=2
  Add3 : Sum
  Constant2 : Constant  Value=0.001
  Divide : Product  Inputs=*/
  Gain : Gain  Gain=1/Ls
  a : Outport
  wires:
  U/1 -> Gain/1
  Divide/1 -> a/1
  w/1 -> Add3/1
  Add3/1 -> Divide/2
  Constant2/1 -> Add3/2
  Gain/1 -> Divide/1

== system dq_model/Tehnika B/Regulacija navora/Limita q toka/napetostna limita/b ==
  U : Inport
  w : Inport  Port=2
  Add4 : Sum
  Constant4 : Constant  Value=0.001
  Divide1 : Product  Inputs=*/
  Gain : Gain  Gain=1/Lst
  b : Outport
  wires:
  Gain/1 -> Divide1/1
  U/1 -> Gain/1
  Constant4/1 -> Add4/2
  Add4/1 -> Divide1/2
  w/1 -> Add4/1
  Divide1/1 -> b/1

== system dq_model/Tehnika s/Regulacija navora/Limita q toka/napetostna limita/a ==
  w : Inport
  U : Inport  Port=2
  Add3 : Sum
  Constant2 : Constant  Value=0.001
  Divide : Product  Inputs=*/
  Gain : Gain  Gain=1/Ls
  a : Outport
  wires:
  U/1 -> Gain/1
  Divide/1 -> a/1
  w/1 -> Add3/1
  Add3/1 -> Divide/2
  Constant2/1 -> Add3/2
  Gain/1 -> Divide/1

== system dq_model/Tehnika s/Regulacija navora/Limita q toka/napetostna limita/b ==
  U : Inport
  w : Inport  Port=2
  Add4 : Sum
  Constant4 : Constant  Value=0.001
  Divide1 : Product  Inputs=*/
  Gain : Gain  Gain=1/Lst
  b : Outport
  wires:
  Gain/1 -> Divide1/1
  U/1 -> Gain/1
  Constant4/1 -> Add4/2
  Add4/1 -> Divide1/2
  w/1 -> Add4/1
  Divide1/1 -> b/1
